simulink model "Sim2016"  (R2016b)
settings: Solver=ode45  StartTime=0.0  StopTime=86400  FixedStep=0.02  RelTol=1e-3
values from neighbouring files (symbols this model uses):
  Mm = 0.02*[1 1 1]    [main.m]
  T0 = [2022 177 0.60599694]    [main.m]
libraries: aerolibgravity2 x1
settings Model: Creator=11986  LastModifiedBy=DSY
settings DataIOCC: ReturnWorkspaceOutputs=on
settings DebuggingCC: SFMachineParentedDataDiag=error
settings SFSimCC: SimUseLocalCustomCode=on
settings RTWCC: RTWUseLocalCustomCode=on

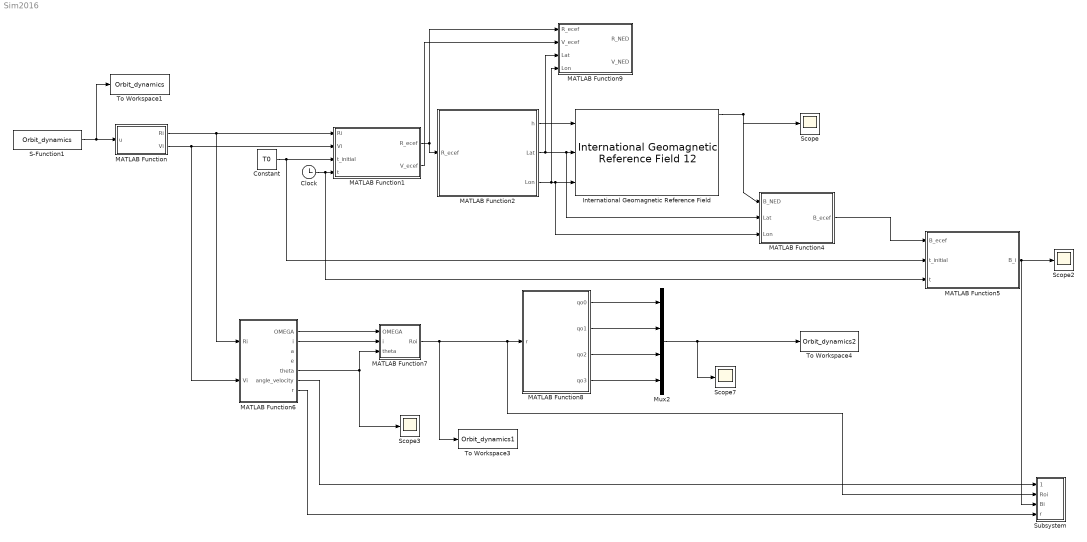
== system Sim2016 ==
  Clock : Clock
  Constant : Constant  Value=T0
  International Geomagnetic Reference Field : aerolibgravity2/International Geomagnetic Reference Field 12  time_in=off  month=June  day=26  year=2022
      settings: AttributesFormatString=%<generation>
  MATLAB Function : MATLAB Function  TreatAsAtomicUnit=on
  MATLAB Function1 : MATLAB Function  TreatAsAtomicUnit=on
  MATLAB Function2 : MATLAB Function  TreatAsAtomicUnit=on
  MATLAB Function4 : MATLAB Function  TreatAsAtomicUnit=on
  MATLAB Function5 : MATLAB Function  TreatAsAtomicUnit=on
  MATLAB Function6 : MATLAB Function  TreatAsAtomicUnit=on
  MATLAB Function7 : MATLAB Function  TreatAsAtomicUnit=on
  MATLAB Function8 : MATLAB Function  TreatAsAtomicUnit=on
  MATLAB Function9 : MATLAB Function  TreatAsAtomicUnit=on
  Mux2 : Mux
  S-Function1 : S-Function  FunctionName=Orbit_dynamics  SFunctionDeploymentMode=off  EnableBusSupport=off
  Scope{,2..3,7} (4 alike) : Scope
  Subsystem : Subsystem
  To Workspace1 : ToWorkspace  VariableName=Orbit_dynamics  SampleTime=-1
  To Workspace3 : ToWorkspace  VariableName=Orbit_dynamics1  SampleTime=-1
  To Workspace4 : ToWorkspace  VariableName=Orbit_dynamics2  SampleTime=-1
  wires:
  S-Function1/1 -> To Workspace1/1, MATLAB Function/1(u)
  Clock/1 -> MATLAB Function5/3(t), MATLAB Function1/4(t)
  MATLAB Function/1(Ri) -> MATLAB Function6/1(Ri), MATLAB Function1/1(Ri)
  Constant/1 -> MATLAB Function5/2(t_initial), MATLAB Function1/3(t_initial)
  MATLAB Function1/1(R_ecef) -> MATLAB Function9/1(R_ecef), MATLAB Function2/1(R_ecef)
  MATLAB Function2/1(h) -> International Geomagnetic Reference Field/1
  MATLAB Function2/3(Lon) -> MATLAB Function4/3(Lon), International Geomagnetic Reference Field/3, MATLAB Function9/4(Lon)
  MATLAB Function2/2(Lat) -> MATLAB Function4/2(Lat), International Geomagnetic Reference Field/2, MATLAB Function9/3(Lat)
  International Geomagnetic Reference Field/1 -> MATLAB Function4/1(B_NED), Scope/1
  MATLAB Function4/1(B_ecef) -> MATLAB Function5/1(B_ecef)
  MATLAB Function5/1(B_i) -> Subsystem/3(Bi), Scope2/1
  MATLAB Function/2(Vi) -> MATLAB Function6/2(Vi), MATLAB Function1/2(Vi)
  MATLAB Function6/2(i) -> MATLAB Function7/2(i)
  MATLAB Function6/5(theta) -> Scope3/1, MATLAB Function7/3(theta)
  MATLAB Function7/1(Roi) -> To Workspace3/1, Subsystem/2(Roi), MATLAB Function8/1(r)
  MATLAB Function6/1(OMEGA) -> MATLAB Function7/1(OMEGA)
  MATLAB Function6/6(angle_velocity) -> Subsystem/1(Angle_velocity)
  MATLAB Function8/1(qo0) -> Mux2/1
  MATLAB Function8/2(qo1) -> Mux2/2
  MATLAB Function8/3(qo2) -> Mux2/3
  MATLAB Function8/4(qo3) -> Mux2/4
  Mux2/1 -> Scope7/1, To Workspace4/1
  MATLAB Function1/2(V_ecef) -> MATLAB Function9/2(V_ecef)
  MATLAB Function6/7(r) -> Subsystem/4(r)

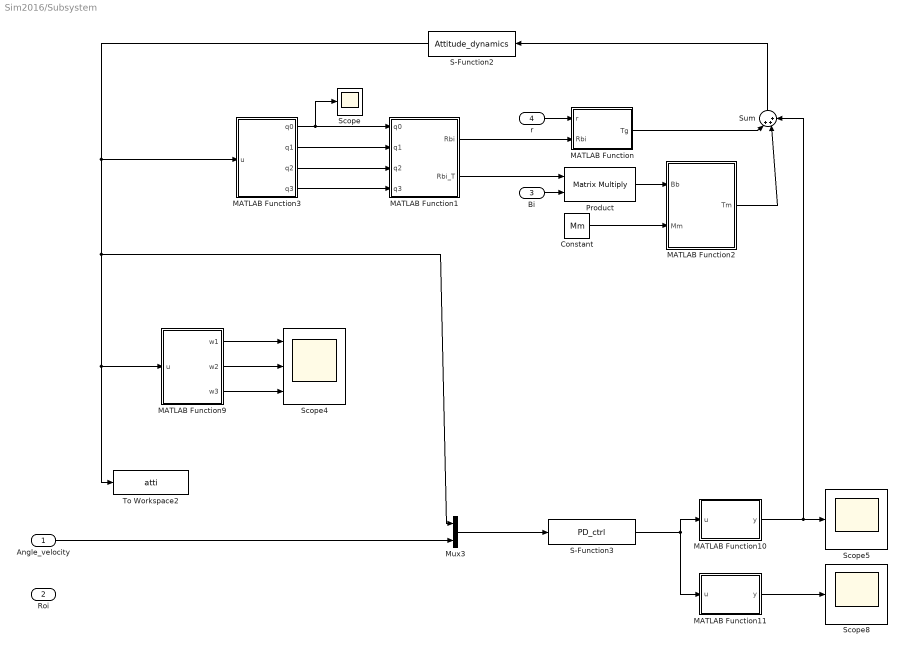
== system Sim2016/Subsystem ==
  Angle_velocity : Inport
  Roi : Inport  Port=2
  Bi : Inport  Port=3
  r : Inport  Port=4
  Constant : Constant  Value=Mm
  MATLAB Function : MATLAB Function  TreatAsAtomicUnit=on
  MATLAB Function1 : MATLAB Function  TreatAsAtomicUnit=on
  MATLAB Function10 : MATLAB Function  TreatAsAtomicUnit=on
  MATLAB Function11 : MATLAB Function  TreatAsAtomicUnit=on
  MATLAB Function2 : MATLAB Function  TreatAsAtomicUnit=on
  MATLAB Function3 : MATLAB Function  TreatAsAtomicUnit=on
  MATLAB Function9 : MATLAB Function  TreatAsAtomicUnit=on
  Mux3 : Mux  Inputs=2
  Product : Product  Multiplication=Matrix(*)
  S-Function2 : S-Function  FunctionName=Attitude_dynamics  SFunctionDeploymentMode=off  EnableBusSupport=off
  S-Function3 : S-Function  FunctionName=PD_ctrl  SFunctionDeploymentMode=off  EnableBusSupport=off
  Scope : Scope
  Scope4 : Scope  NumInputPorts=3
  Scope5 : Scope
  Scope8 : Scope
  Sum : Sum  Inputs=|+++
  To Workspace2 : ToWorkspace  VariableName=atti  SampleTime=-1
  wires:
  MATLAB Function3/1(q0) -> MATLAB Function1/1(q0), Scope/1
  MATLAB Function10/1(y) -> Sum/3, Scope5/1
  MATLAB Function3/2(q1) -> MATLAB Function1/2(q1)
  MATLAB Function9/3(w3) -> Scope4/3
  MATLAB Function3/3(q2) -> MATLAB Function1/3(q2)
  S-Function2/1 -> Mux3/1, MATLAB Function9/1(u), To Workspace2/1, MATLAB Function3/1(u)
  MATLAB Function3/4(q3) -> MATLAB Function1/4(q3)
  MATLAB Function11/1(y) -> Scope8/1
  S-Function3/1 -> MATLAB Function10/1(u), MATLAB Function11/1(u)
  MATLAB Function9/1(w1) -> Scope4/1
  Mux3/1 -> S-Function3/1
  MATLAB Function9/2(w2) -> Scope4/2
  Angle_velocity/1 -> Mux3/2
  MATLAB Function1/2(Rbi_T) -> Product/1
  Bi/1 -> Product/2
  Product/1 -> MATLAB Function2/1(Bb)
  r/1 -> MATLAB Function/1(r)
  MATLAB Function1/1(Rbi) -> MATLAB Function/2(Rbi)
  Constant/1 -> MATLAB Function2/2(Mm)
  MATLAB Function2/1(Tm) -> Sum/2
  MATLAB Function/1(Tg) -> Sum/1
  Sum/1 -> S-Function2/1

== matlab function Sim2016/MATLAB Function1 ==
  data: Ri input; Vi input; R_ecef output; t_initial input; t input; V_ecef output
function [R_ecef,V_ecef] = ECI2ECEF(Ri,Vi,t_initial,t)

% utc=UTC_cal(2022,177,0.60599694,t);
% jd=UTC2JD(utc);
y=2.459757105996940e+06/36525;

theta_g0=(24110.54841+8640184.812866*y+0.093104*y^2-6.2e-6*y^3);
omega_e=7.2921151e-5;
theta_g=theta_g0+omega_e*t;

R_ecef=Rotatez(theta_g)'*Ri;
V_ecef=Rotatez(theta_g)'*Vi;

== matlab function Sim2016/MATLAB Function ==
  data: u input; Ri output; Vi output
function [Ri,Vi] = fcn(u)

Ri=[u(1),u(2),u(3)]';
Vi =[u(4),u(5),u(6)]';

== matlab function Sim2016/MATLAB Function2 ==
  data: R_ecef input; h output; Lat output; Lon output
function [h,Lat,Lon] = Cartesian2LL(R_ecef)

h=sqrt(R_ecef'*R_ecef);

angle=atan(R_ecef(2)/R_ecef(1));
if R_ecef(1)>=0
    Lon=angle;
elseif R_ecef(1)<0&&angle>0
    Lon=angle-pi;
elseif R_ecef(1)<0&&angle<0
    Lon=angle+pi;
else
    Lon=0
end
Lat=atan(R_ecef(3)/h);

Lat=Lat*180/2/pi;
Lon=Lon*180/2/pi;

== matlab function Sim2016/Subsystem/MATLAB Function3 ==
  data: u input; q0 output; q1 output; q2 output; q3 output
function [q0,q1,q2,q3] = fcn(u)

q0=u(1)
q1=u(2)
q2=u(3)
q3=u(4)

== matlab function Sim2016/MATLAB Function4 ==
  data: B_NED input; B_ecef output; Lat input; Lon input
function B_ecef = fcn(B_NED,Lat,Lon)

B_ecef=Rotatez(Lon/180*pi)*Rotatey(-(Lat+90)/180*pi)*B_NED;

== matlab function Sim2016/MATLAB Function5 ==
  data: B_ecef input; B_i output; t_initial input; t input
function B_i = ECEF2ECI(B_ecef,t_initial,t)

% utc=UTC_cal(2022,177,0.60599694,t);
% jd=UTC2JD(utc);
y=2.459757105996940e+06/36525;

theta_g0=(24110.54841+8640184.812866*y+0.093104*y^2-6.2e-6*y^3);
omega_e=7.2921151e-5;
theta_g=theta_g0+omega_e*t;


B_i=Rotatez(theta_g)*B_ecef;

== matlab function Sim2016/MATLAB Function6 ==
  data: Ri input; OMEGA output; Vi input; i output; a output; e output; theta output; angle_velocity output; r output
function [OMEGA,i,a,e,theta,angle_velocity,r] = fcn(Ri,Vi)
uE = 3.986004418e+5;

x=Ri(1);
y=Ri(2);
z=Ri(3);
x_dot=Vi(1);
y_dot=Vi(2);
z_dot=Vi(3);

r=sqrt(x^2+y^2+z^2);%%%半径
v=sqrt(x_dot^2+y_dot^2+z_dot^2);%%%速度
a=1/(2/r-(x_dot^2+y_dot^2+z_dot^2)/uE);%%%半长轴
h=[0 -z y;z 0 -x;-y x 0]*Vi;%%%角动量
p=h'*h/uE;%%%半通径
e=sqrt(1-p/a);%%%离心率

i=acos(h(3)/sqrt(h'*h));%%%
vec_N=[0 -1 0;1 0 0;0 0 0]*h%%%节线方向;
BIG_OMEGA=acos(vec_N(1)/sqrt(vec_N'*vec_N));%%%升交点赤经
theta=acos(vec_N'*Ri/sqrt(vec_N'*vec_N)/r);%%%升交点幅角
% f=acos((p-r)/r/e);%%%真近角
% little_omega=theta-f;%%%近地点幅角

OMEGA=BIG_OMEGA;
angle_velocity=[0;-sqrt(h'*h)/r^2;0];
% omega=little_omega;

== matlab function Sim2016/MATLAB Function7 ==
  data: OMEGA input; Roi output; i input; theta input
function Roi = fcn(OMEGA,i,theta)
%%%轨道坐标系中位置与速度
Roi=Rotatez(OMEGA)*Rotatex(i)*Rotatez(theta+pi/2)*Rotatex(-pi/2);

== matlab function Sim2016/MATLAB Function8 ==
  data: r input; qo0 output; qo1 output; qo2 output; qo3 output
function [qo0,qo1,qo2,qo3]= Matrix2Quaternion(r)

S=haha(r(3,2)-r(2,3))+haha(r(1,3)-r(3,1))+haha((r(2,1)-r(1,2)));
qo0=sqrt(1+r(1,1)+r(2,2)+r(3,3))/2;

if S==1
    qo0=-sqrt(1+r(1,1)+r(2,2)+r(3,3))/2;
elseif S==2||S==0||S==3
    ;
else
end
qo1=(r(3,2)-r(2,3))/4/qo0;
qo2=(r(1,3)-r(3,1))/4/qo0;
qo3=(r(2,1)-r(1,2))/4/qo0;

end

function score=haha(f)
if f>0
    score=1;
else
    score=0;
end
end

== matlab function Sim2016/Subsystem/MATLAB Function9 ==
  data: u input; w1 output; w2 output; w3 output
function [w1,w2,w3] = fcn(u)

w1=u(5)
w2=u(6)
w3=u(7)

== matlab function Sim2016/Subsystem/MATLAB Function10 ==
  data: u input; y output
function y = fcn(u)

y = u(1:3);

== matlab function Sim2016/Subsystem/MATLAB Function11 ==
  data: u input; y output
function y = fcn(u)

y = u(8:11);

== matlab function Sim2016/Subsystem/MATLAB Function1 ==
  data: q0 input; Rbi output; q1 input; q2 input; q3 input; Rbi_T output
function [Rbi,Rbi_T]  = fcn(q0,q1,q2,q3)

Rbi=[1-2*q2^2-2*q3^2 2*q1*q2-2*q0*q3 2*q1*q3+2*q0*q2;
    2*q1*q2+2*q0*q3 1-2*q1^2-2*q3^2 2*q2*q3-2*q0*q1;
    2*q1*q3-2*q0*q2 2*q2*q3+2*q0*q1 1-2*q1*2-2*q2^2];
Rbi_T=Rbi';

== matlab function Sim2016/MATLAB Function9 ==
  data: R_ecef input; V_ecef input; R_NED output; Lat input; Lon input; V_NED output
function [R_NED,V_NED] = fcn(R_ecef,V_ecef,Lat,Lon)


R_NED=Rotatey(-(Lat+90)/180*pi)'*Rotatez(Lon/180*pi)'*R_ecef;
V_NED=Rotatey(-(Lat+90)/180*pi)'*Rotatez(Lon/180*pi)'*V_ecef;

== matlab function Sim2016/Subsystem/MATLAB Function ==
  data: r input; Rbi input; Tg output
function Tg = fcn(r,Rbi)
J=[7.659 -0.002 0.038;
    -0.002 7.6490 -0.0170;
    0.038 -0.017 0.5330];

E=Rbi*[0;0;1];
uE = 3.986004418e+5;

EX=[0 -E(3) E(2);E(3) 0 -E(1);-E(2) E(1) 0];

Tg=-3*uE/r^3*(EX*J*E);

== matlab function Sim2016/Subsystem/MATLAB Function2 ==
  data: Bb input; Mm input; Tm output
function Tm = fcn(Bb,Mm)




MmX=[0 -Mm(3) Mm(2);Mm(3) 0 -Mm(1);-Mm(2) Mm(1) 0];

Tm=MmX*Bb*10e-9;
